simulink model "quarterCarModelsDomain"  (R2025a)
settings: Solver=VariableStepAuto  StartTime=0.0  StopTime=10.0  RelTol=1e-3
undefined symbols (not defined in the file): c1, k1, k2, mc, ms
settings Model: Creator=krishDragneel  LastModifiedBy=krishDragneel

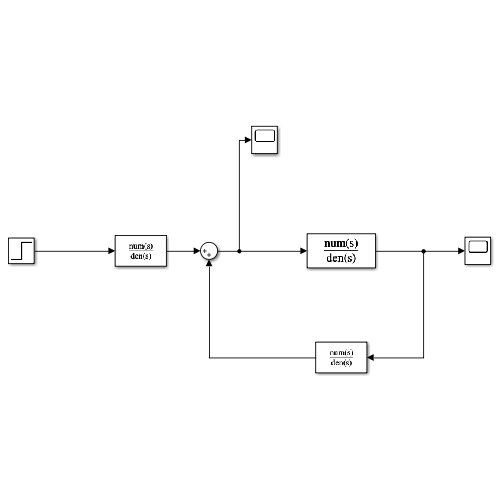
[thumbnail: Simulink's stored preview of the top-level diagram]
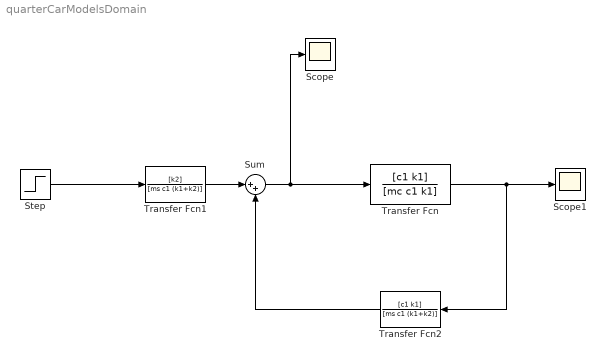
== system quarterCarModelsDomain ==
  Scope : Scope
      settings: ActiveDisplayYMinimum=-0.19377879485462485  ActiveDisplayYMaximum=1.744009153691624
  Scope1 : Scope
      settings: ActiveDisplayYMinimum=-0.17280164838315135  ActiveDisplayYMaximum=1.5552148354483624
  Step : Step  SampleTime=0
  Sum : Sum  Inputs=|++
  Transfer Fcn : TransferFcn  Numerator=[c1 k1]  Denominator=[mc c1 k1]
  Transfer Fcn1 : TransferFcn  Numerator=[k2]  Denominator=[ms c1 (k1+k2)]
  Transfer Fcn2 : TransferFcn  Numerator=[c1 k1]  Denominator=[ms c1 (k1+k2)]
  wires:
  Transfer Fcn/1 -> Transfer Fcn2/1, Scope1/1
  Step/1 -> Transfer Fcn1/1
  Transfer Fcn1/1 -> Sum/1
  Transfer Fcn2/1 -> Sum/2
  Sum/1 -> Scope/1, Transfer Fcn/1
